simulink model "stickman3Rev2022a"  (R2022a)
settings: Solver=VariableStepAuto  StartTime=0.0  StopTime=1.5  RelTol=1e-3
libraries: aerolibanim x1, shared6dof x1
settings Model: PacingRate=0.110000  Creator=mthorbu  LastModifiedBy=matho

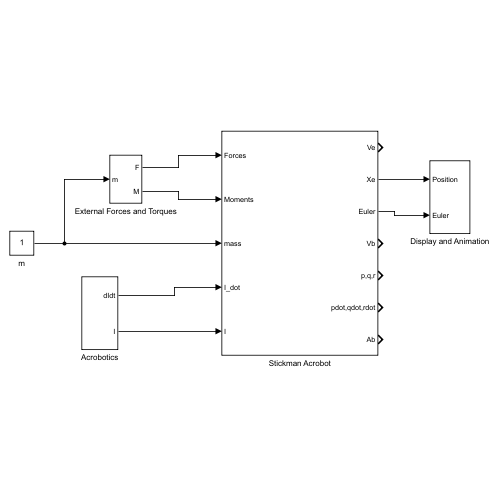
[thumbnail: Simulink's stored preview of the top-level diagram]
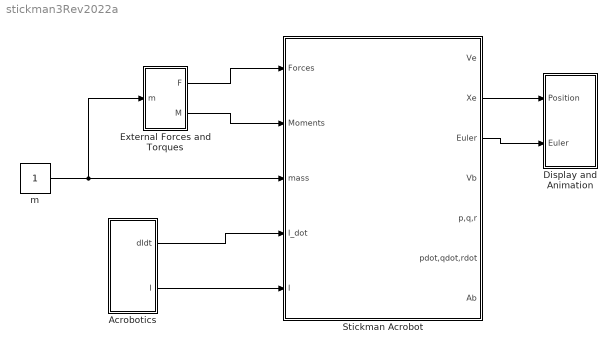
== system stickman3Rev2022a ==
  Acrobotics : Subsystem
  Display and Animation : Subsystem
  External Forces and Torques : Subsystem
  Stickman Acrobot : Subsystem
  m : Constant
  wires:
  m/1 -> External Forces and Torques/1(m), Stickman Acrobot/3(mass)
  External Forces and Torques/1(F) -> Stickman Acrobot/1(Forces)
  External Forces and Torques/2(M) -> Stickman Acrobot/2(Moments)
  Acrobotics/1(dIdt) -> Stickman Acrobot/4(I_dot)
  Acrobotics/2(I) -> Stickman Acrobot/5(I)
  Stickman Acrobot/2(Xe) -> Display and Animation/1(Position)
  Stickman Acrobot/3(Euler) -> Display and Animation/2(Euler)

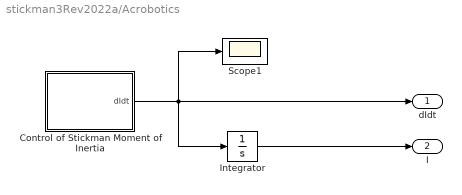
== system stickman3Rev2022a/Acrobotics ==
  Control of Stickman Moment of Inertia : Stateflow chart  TreatAsAtomicUnit=on
  Integrator : Integrator  InitialCondition=eye(3)
  Scope1 : Scope
  dIdt : Outport
  I : Outport  Port=2
  wires:
  Control of Stickman Moment of Inertia/1(dIdt) -> dIdt/1, Scope1/1, Integrator/1
  Integrator/1 -> I/1

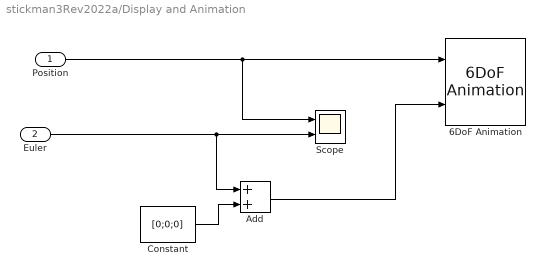
== system stickman3Rev2022a/Display and Animation ==
  Position : Inport
  Euler : Inport  Port=2
  6DoF Animation : aerolibanim/6DoF Animation  u1=[-50 50 -50 50 -100 0]  u2=0.05  u3=3.0  u4=[0,0,0]  u5=Fixed position  u6=[10,10,0]  u7=90  u8=on
  Add : Sum
  Constant : Constant  Value=[0;0;0]
  Scope : Scope  NumInputPorts=2
  wires:
  Euler/1 -> Scope/2, Add/1
  Position/1 -> Scope/1, 6DoF Animation/1
  Constant/1 -> Add/2
  Add/1 -> 6DoF Animation/2

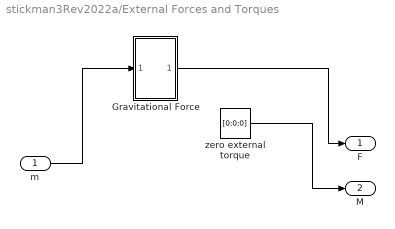
== system stickman3Rev2022a/External Forces and Torques ==
  m : Inport
  Gravitational Force : Subsystem
  zero external torque : Constant  Value=[0;0;0]
  F : Outport
  M : Outport  Port=2
  wires:
  zero external torque/1 -> M/1
  m/1 -> Gravitational Force/1(In1)
  Gravitational Force/1(Out1) -> F/1

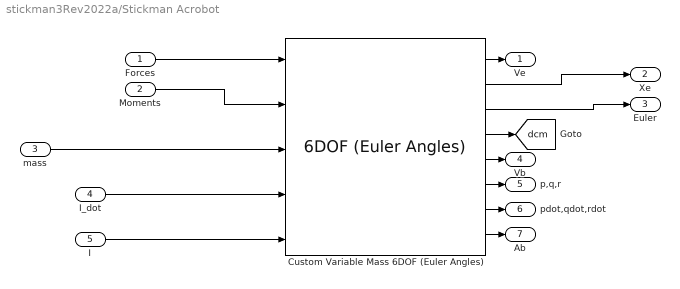
== system stickman3Rev2022a/Stickman Acrobot ==
  Forces : Inport
  Moments : Inport  Port=2
  mass : Inport  Port=3
  I_dot : Inport  Port=4
  I : Inport  Port=5
  Custom Variable Mass 6DOF (Euler Angles) : shared6dof/6DOF (Euler Angles)  units=Metric (MKS)  mtype=Custom Variable  rep=Euler Angles  xme_0="[4  0  -2-4]"  Vm_0=[11 0 0]  eul_0=[0 0 0]  pm_0=[0 0.5 0]  mass_0=1.0  mass_e=0.5  mass_f=2.0  inertia=eye(3)  inertia_e=eye(3)  inertia_f=2*eye(3)  k_quat=1.0  vre_flag=off  abi_flag=off  aMode=0  xme_statename=''  Vm_statename=''  eul_statename=''  quat_statename=''  pm_statename=''  mass_statename=''
  Ve : Outport
  Xe : Outport  Port=2
  Euler : Outport  Port=3
  Vb : Outport  Port=4
  p,q,r : Outport  Port=5
  pdot,qdot,rdot : Outport  Port=6
  Ab : Outport  Port=7
  tag scope: dcm=global
  wires:
  Custom Variable Mass 6DOF (Euler Angles)/6 -> p,q,r/1
  Moments/1 -> Custom Variable Mass 6DOF (Euler Angles)/2
  Custom Variable Mass 6DOF (Euler Angles)/1 -> Ve/1
  Custom Variable Mass 6DOF (Euler Angles)/4 -> [dcm]
  Forces/1 -> Custom Variable Mass 6DOF (Euler Angles)/1
  Custom Variable Mass 6DOF (Euler Angles)/3 -> Euler/1
  I_dot/1 -> Custom Variable Mass 6DOF (Euler Angles)/4
  Custom Variable Mass 6DOF (Euler Angles)/2 -> Xe/1
  Custom Variable Mass 6DOF (Euler Angles)/5 -> Vb/1
  I/1 -> Custom Variable Mass 6DOF (Euler Angles)/5
  Custom Variable Mass 6DOF (Euler Angles)/7 -> pdot,qdot,rdot/1
  Custom Variable Mass 6DOF (Euler Angles)/8 -> Ab/1
  mass/1 -> Custom Variable Mass 6DOF (Euler Angles)/3

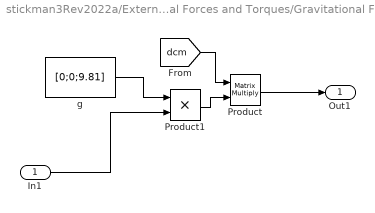
== system stickman3Rev2022a/External Forces and Torques/Gravitational Force ==
  In1 : Inport
  Product : Product  Multiplication=Matrix(*)
  Product1 : Product
  g : Constant  Value=[0;0;9.81]
  Out1 : Outport
  wires:
  [dcm] -> Product/1
  g/1 -> Product1/1
  Product1/1 -> Product/2
  Product/1 -> Out1/1
  In1/1 -> Product1/2

== stateflow chart stickman3Rev2022a/Acrobotics/Control of Stickman Moment of Inertia ==
  state Initialize
    entry:
    dIdt=0*eye(3);
  state transiton
    entry:
    dIdt=-8*eye(3);
  state transiton2
    entry:
    dIdt=0*eye(3);
  (default) -> Initialize
  Initialize -> transiton : [after(0.2,sec)]
  transiton -> transiton2 : [after(0.1,sec)]
  data: dIdt output
